simulink model "dofAutopilot"  (R2024b)
settings: Solver=ode4  StartTime=0.0  StopTime=10  FixedStep=0.001  MaxStep=0.2  RelTol=1e-3
libraries: slpidlib x2, shared6dof x1, aerolibatmos2 x1
settings Model: Creator=sahil  LastModifiedBy=sahil

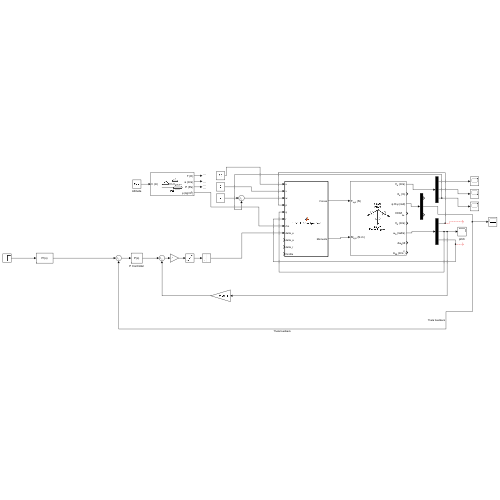
[thumbnail: Simulink's stored preview of the top-level diagram]
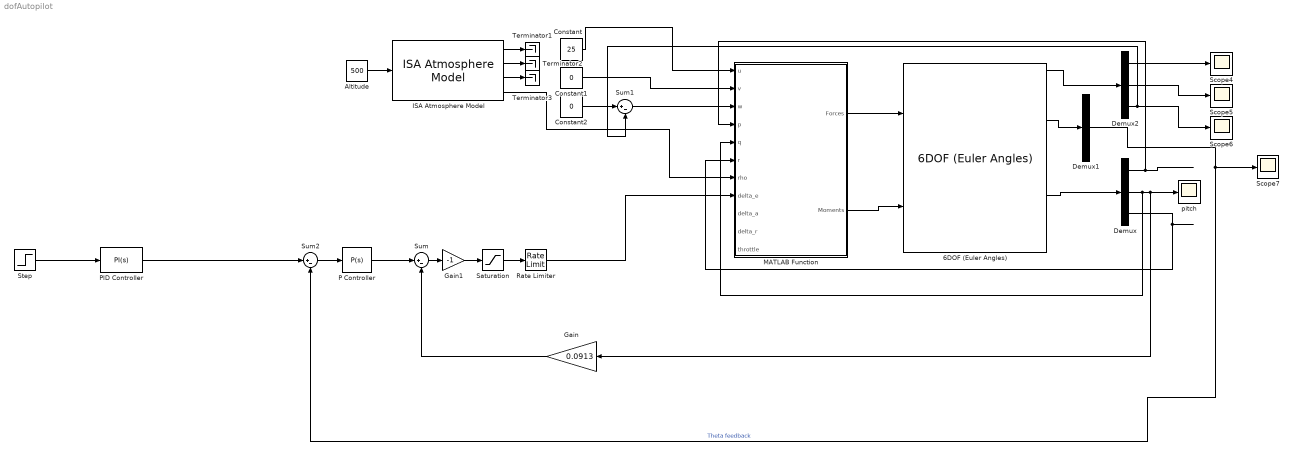
== system dofAutopilot ==
  6DOF (Euler Angles) : shared6dof/6DOF (Euler Angles)  units=Metric (MKS)  mtype=Fixed  rep=Euler Angles  xme_0=[0 0 0]  Vm_0=[15 0 0]  eul_0=[0 0 0]  pm_0=[0 0 0]  mass_0=13.5  mass_e=0.5  mass_f=2.0  inertia=[0.824 0 0.120; 0 1.135 0; 0.120 0 1.759]  inertia_e=eye(3)  inertia_f=2*eye(3)  k_quat=1.0  vre_flag=on  abi_flag=off  aMode=0  xme_statename=''  Vm_statename=''  eul_statename=''  quat_statename=''  pm_statename=''  mass_statename=''
  Altitude : Constant  Value=500
  Constant : Constant  Value=25
  Constant1 : Constant  Value=0
  Constant2 : Constant  Value=0
  Demux : Demux  Outputs=3
  Demux1 : Demux  Outputs=3
  Demux2 : Demux  Outputs=3
  Gain : Gain  Gain=0.0913
  Gain1 : Gain  Gain=-1
  ISA Atmosphere Model : aerolibatmos2/ISA Atmosphere Model  useExtended=off  action=Warning  custom=off  viscosityOut=off  g=9.80665  gamma=1.4  R=287.0531  L=0.0065  h_trop=11000  h_strat=20000  rho0=1.225  P0=101325  T0=288.15  h0=0  S=110.4  Tref=273.15  muref=1.716e-5
  MATLAB Function : MATLAB Function  TreatAsAtomicUnit=on
  P Controller : slpidlib/PID Controller  Controller=P  Form=Parallel  TimeDomain=Continuous-time  UseExternalTs=off  SampleTime=-1  IntegratorMethod=Forward Euler  FilterMethod=Forward Euler  ControllerParametersSource=internal  P=1.01058981940052  I=0  UseKiTs=off  D=0  UseExternalDerivativeSource=off  N=100  UseFilter=on  TunerSelectOption=Transfer Function Based (PID Tuner App)  InitialConditionSource=internal  InitialConditionForIntegrator=0  InitialConditionForFilter=0  DifferentiatorICPrevScaledInput=0  ExternalReset=none  TrackingMode=off  Kt=1  LimitOutput=off  SatLimitsSource=internal  UpperSaturationLimit=inf  LowerSaturationLimit=-inf  LinearizeAsGain=on  AntiWindupMode=none  Kb=1  LimitIntegrator=off  UpperIntegratorSaturationLimit=inf  LowerIntegratorSaturationLimit=-inf  POutMin=[]  POutMax=[]  IOutMin=[]  IOutMax=[]  DOutMin=[]  DOutMax=[]  NOutMin=[]  NOutMax=[]  SumOutMin=[]  SumOutMax=[]  SaturationOutMin=[]  SaturationOutMax=[]  PParamMin=[]  PParamMax=[]  IParamMin=[]  IParamMax=[]  DParamMin=[]  DParamMax=[]  NParamMin=[]  NParamMax=[]  KbParamMin=[]  KbParamMax=[]  KtParamMin=[]  KtParamMax=[]  KbOutMin=[]  KbOutMax=[]  KtOutMin=[]  KtOutMax=[]  IntegratorOutMin=[]  IntegratorOutMax=[]  FilterOutMin=[]  FilterOutMax=[]  SumI1OutMin=[]  SumI1OutMax=[]  SumI2OutMin=[]  SumI2OutMax=[]  SumI3OutMin=[]  SumI3OutMax=[]  SumI4OutMin=[]  SumI4OutMax=[]  SumDOutMin=[]  SumDOutMax=[]  DifferentiatorOutMin=[]  DifferentiatorOutMax=[]  FilterDiffOutCoefMin=[]  FilterDiffOutCoefMax=[]  ReciprocalOutMin=[]  ReciprocalOutMax=[]  SumDenOutMin=[]  SumDenOutMax=[]  SumNumOutMin=[]  SumNumOutMax=[]  DivideOutMin=[]  DivideOutMax=[]  UdiffTsProdOutMin=[]  UdiffTsProdOutMax=[]  NTsProdOutMin=[]  NTsProdOutMax=[]  UintegralTsProdOutMin=[]  UintegralTsProdOutMax=[]  UngainTsProdOutMin=[]  UngainTsProdOutMax=[]  ClampingZeroOutDataTypeStr=Inherit: Inherit via back propagation  ClampingZeroOutMin=[]  ClampingZeroOutMax=[]  FilterDenConstantOutDataTypeStr=Inherit: Inherit via back propagation  FilterDenConstantOutMin=[]  FilterDenConstantOutMax=[]  PCopyOutDataTypeStr=Inherit: Inherit via back propagation  PCopyOutMin=[]  PCopyOutMax=[]  NCopyOutDataTypeStr=Inherit: Inherit via back propagation  NCopyOutMin=[]  NCopyOutMax=[]  IntegratorContinuousStateAttributes=''  IntegratorStateMustResolveToSignalObject=off  IntegratorRTWStateStorageClass=Auto  FilterContinuousStateAttributes=''  FilterStateMustResolveToSignalObject=off  FilterRTWStateStorageClass=Auto  ParallelPVariant=InternalParameters  IdealPVariant=Disabled  IVariant=Disabled  DVariant=Disabled  IntegratorVariant=Disabled  SatVariant=Disabled  AWVariant=Disabled  PCopyVariant=Disabled  TRVariant=Disabled  FdbkBlocksVariant=Forward  IdealPFdbkVariant=Disabled  SatFdbkVariant=Disabled  DerivativeFilterVariant=Disabled  NVariant=Disabled  NCopyVariant=Disabled_SignalSpec  FilterICVariant=Disabled  IntegratorICVariant=Disabled  ExternalResetVariant=Disabled  TRSumVariant=Passthrough  SumFdbkVariant=Disabled  SumVariant=Passthrough_P  TsampFilterVariant=InternalTs  TsampNgainVariant=Passthrough  TsampIntegralVariant=Disabled_SignalSpec  ExternalSaturationOutDataTypeStr=Inherit: Same as second input  DerivativeSourceVariant=Disabled  PreIntVariant=InternalPreInt
  PID Controller : slpidlib/PID Controller  Controller=PI  Form=Parallel  TimeDomain=Continuous-time  UseExternalTs=off  SampleTime=-1  IntegratorMethod=Forward Euler  FilterMethod=Forward Euler  ControllerParametersSource=internal  P=0.00302835474355919  I=0.00038250519229473  UseKiTs=off  D=0  UseExternalDerivativeSource=off  N=100  UseFilter=on  TunerSelectOption=Transfer Function Based (PID Tuner App)  InitialConditionSource=internal  InitialConditionForIntegrator=0  InitialConditionForFilter=0  DifferentiatorICPrevScaledInput=0  ExternalReset=none  TrackingMode=off  Kt=1  LimitOutput=off  SatLimitsSource=internal  UpperSaturationLimit=inf  LowerSaturationLimit=-inf  LinearizeAsGain=on  AntiWindupMode=none  Kb=1  LimitIntegrator=off  UpperIntegratorSaturationLimit=inf  LowerIntegratorSaturationLimit=-inf  POutMin=[]  POutMax=[]  IOutMin=[]  IOutMax=[]  DOutMin=[]  DOutMax=[]  NOutMin=[]  NOutMax=[]  SumOutMin=[]  SumOutMax=[]  SaturationOutMin=[]  SaturationOutMax=[]  PParamMin=[]  PParamMax=[]  IParamMin=[]  IParamMax=[]  DParamMin=[]  DParamMax=[]  NParamMin=[]  NParamMax=[]  KbParamMin=[]  KbParamMax=[]  KtParamMin=[]  KtParamMax=[]  KbOutMin=[]  KbOutMax=[]  KtOutMin=[]  KtOutMax=[]  IntegratorOutMin=[]  IntegratorOutMax=[]  FilterOutMin=[]  FilterOutMax=[]  SumI1OutMin=[]  SumI1OutMax=[]  SumI2OutMin=[]  SumI2OutMax=[]  SumI3OutMin=[]  SumI3OutMax=[]  SumI4OutMin=[]  SumI4OutMax=[]  SumDOutMin=[]  SumDOutMax=[]  DifferentiatorOutMin=[]  DifferentiatorOutMax=[]  FilterDiffOutCoefMin=[]  FilterDiffOutCoefMax=[]  ReciprocalOutMin=[]  ReciprocalOutMax=[]  SumDenOutMin=[]  SumDenOutMax=[]  SumNumOutMin=[]  SumNumOutMax=[]  DivideOutMin=[]  DivideOutMax=[]  UdiffTsProdOutMin=[]  UdiffTsProdOutMax=[]  NTsProdOutMin=[]  NTsProdOutMax=[]  UintegralTsProdOutMin=[]  UintegralTsProdOutMax=[]  UngainTsProdOutMin=[]  UngainTsProdOutMax=[]  ClampingZeroOutDataTypeStr=Inherit: Inherit via back propagation  ClampingZeroOutMin=[]  ClampingZeroOutMax=[]  FilterDenConstantOutDataTypeStr=Inherit: Inherit via back propagation  FilterDenConstantOutMin=[]  FilterDenConstantOutMax=[]  PCopyOutDataTypeStr=Inherit: Inherit via back propagation  PCopyOutMin=[]  PCopyOutMax=[]  NCopyOutDataTypeStr=Inherit: Inherit via back propagation  NCopyOutMin=[]  NCopyOutMax=[]  IntegratorContinuousStateAttributes=''  IntegratorStateMustResolveToSignalObject=off  IntegratorRTWStateStorageClass=Auto  FilterContinuousStateAttributes=''  FilterStateMustResolveToSignalObject=off  FilterRTWStateStorageClass=Auto  ParallelPVariant=InternalParameters  IdealPVariant=Disabled  IVariant=InternalParameters  DVariant=Disabled  IntegratorVariant=Continuous  SatVariant=Disabled  AWVariant=Passthrough  PCopyVariant=Disabled  TRVariant=Disabled  FdbkBlocksVariant=Forward  IdealPFdbkVariant=Disabled  SatFdbkVariant=Disabled  DerivativeFilterVariant=Disabled  NVariant=Disabled  NCopyVariant=Disabled_SignalSpec  FilterICVariant=Disabled  IntegratorICVariant=InternalICs  ExternalResetVariant=Disabled  TRSumVariant=Passthrough  SumFdbkVariant=Disabled  SumVariant=Sum_PI  TsampFilterVariant=InternalTs  TsampNgainVariant=Passthrough  TsampIntegralVariant=Disabled_SignalSpec  ExternalSaturationOutDataTypeStr=Inherit: Same as second input  DerivativeSourceVariant=Disabled  PreIntVariant=InternalPreInt
  Rate Limiter : RateLimiter  RisingSlewLimit=45*pi/180  FallingSlewLimit=-45*pi/180  SampleTimeMode=inherited
  Saturation : Saturate  UpperLimit=25*pi/180  LowerLimit=-25*pi/180
  Scope{4..7} (4 alike) : Scope
  Step : Step  After=5/57.3  SampleTime=0
  Sum : Sum  Inputs=|+-
  Sum1 : Sum  Inputs=|+-
  Sum2 : Sum  Inputs=|+-
  Terminator1 : Terminator
  Terminator2 : Terminator
  Terminator3 : Terminator
  pitch : Scope
  wires:
  Altitude/1 -> ISA Atmosphere Model/1
  ISA Atmosphere Model/1 -> Terminator1/1
  ISA Atmosphere Model/2 -> Terminator2/1
  ISA Atmosphere Model/3 -> Terminator3/1
  ISA Atmosphere Model/4 -> MATLAB Function/7(rho)
  MATLAB Function/1(Forces) -> 6DOF (Euler Angles)/1
  MATLAB Function/2(Moments) -> 6DOF (Euler Angles)/2
  6DOF (Euler Angles)/1 -> Demux2/1
  6DOF (Euler Angles)/6 -> Demux/1
  Demux/1 -> MATLAB Function/4(p)
  Demux/3 -> MATLAB Function/6(r)
  Demux2/1 -> Scope4/1
  Demux2/2 -> Scope5/1
  Demux2/3 -> Sum1/2, Scope6/1
  Constant/1 -> MATLAB Function/1(u)
  Constant1/1 -> MATLAB Function/2(v)
  Constant2/1 -> Sum1/1
  Sum1/1 -> MATLAB Function/3(w)
  6DOF (Euler Angles)/3 -> Demux1/1
  Gain1/1 -> Saturation/1
  PID Controller/1 -> Sum2/1
  Step/1 -> PID Controller/1
  Saturation/1 -> Rate Limiter/1
  Sum/1 -> Gain1/1
  Gain/1 -> Sum/2
  Rate Limiter/1 -> MATLAB Function/8(delta_e)
  Sum2/1 -> P Controller/1
  Demux1/2 -> Sum2/2, Scope7/1  "Theta feedback"
  P Controller/1 -> Sum/1
  Demux/2 -> MATLAB Function/5(q), Gain/1, pitch/1

== matlab function dofAutopilot/MATLAB Function ==
  data: u input; Forces output; v input; w input; p input; q input; r input; rho input; Moments output; delta_e input; delta_a input; delta_r input; throttle input
function [Forces, Moments] = computeAeroDynamics(u, v, w, p, q, r, rho, delta_e, delta_a, delta_r, throttle)
% Inputs:
% u, v, w  - Body frame velocities in m/s
% p, q, r  - Body frame angular rates in rad/s
% rho      - Air density in kg/m^3
% delta_e  - Elevator deflection in radians
% delta_a  - Aileron deflection in radians
% delta_r  - Rudder deflection in radians
% throttle - Throttle command (0 to 1)

    %% 1. Aircraft Geometry & Reference Values (Aerosonde UAV)
    S = 0.55;         % Reference wing area (m^2)
    b = 2.895;        % Wingspan (m)
    c_bar = 0.1899;   % Mean aerodynamic chord (m)
    
    %% 2. Airflow Angles & Dynamic Pressure
    V = sqrt(u^2 + v^2 + w^2);
    V_safe = max(V, 0.1); 
    
    alpha = atan2(w, u);
    beta = asin(v / V_safe);
    
    q_bar = 0.5 * rho * V^2; % Dynamic pressure
    
    %% 3. Aerodynamic Stability Derivatives (Aerosonde Standards)
    % Longitudinal Derivatives
    CL0 = 0.28;      CLa = 5.61;      CLq = 0;      CLde = 0.13;
    CD0 = 0.03;      K = 0.055;       % Induced drag factor
    Cm0 = -0.02;     Cma = -2.74;     Cmq = -38.21;    Cmde = -2.31; % FIXED: Was -231
    
    % Lateral-Directional Derivatives
    CYb = -0.17;     CYp = 0;         CYr = 0;         CYdr = 0.208;
    Clb = -0.13;     Clp = -0.51;     Clr = 0.265;     Clda = 0.17;   Cldr = 0.045;
    Cnb = 0.073;     Cnp = -0.14;     Cnr = -0.096;    Cnda = 0.0042;  Cndr = -0.069;
    
    %% 4. Non-Dimensional Coefficients
    % Lift, Drag, and Pitch Moment
    CL = CL0 + CLa*alpha + CLq*(q*c_bar/(2*V_safe)) + CLde*delta_e;
    CD = CD0 + K*(CL^2);
    Cm = Cm0 + Cma*alpha + Cmq*(q*c_bar/(2*V_safe)) + Cmde*delta_e;
    
    % Sideforce, Roll, and Yaw Moment
    CY = CYb*beta + CYp*(p*b/(2*V_safe)) + CYr*(r*b/(2*V_safe)) + CYdr*delta_r;
    Cl = Clb*beta + Clp*(p*b/(2*V_safe)) + Clr*(r*b/(2*V_safe)) + Clda*delta_a + Cldr*delta_r;
    Cn = Cnb*beta + Cnp*(p*b/(2*V_safe)) + Cnr*(r*b/(2*V_safe)) + Cnda*delta_a + Cndr*delta_r;
    
    %% 5. Dimensional Aerodynamic Forces (Wind to Body Frame)
    L_aero = q_bar * S * CL;
    D_aero = q_bar * S * CD;
    Y_aero = q_bar * S * CY;
    
    Fx_aero = -D_aero * cos(alpha) + L_aero * sin(alpha);
    Fy_aero = Y_aero;
    Fz_aero = -D_aero * sin(alpha) - L_aero * cos(alpha);
    
    %% 6. Dimensional Aerodynamic Moments
    L_moment = q_bar * S * b * Cl;
    M_moment = q_bar * S * c_bar * Cm;
    N_moment = q_bar * S * b * Cn;
    
    %% 7. Propulsion Model
    % Realistic thrust for a 13.5kg UAV (approx 80N max)
    max_thrust = 80; 
    Thrust = max_thrust * throttle;
    
    Fx_total = Fx_aero + Thrust;
    Fy_total = Fy_aero;
    Fz_total = Fz_aero;
    
    %% 8. Compile Outputs
    Forces = [Fx_total; Fy_total; Fz_total];
    Moments = [L_moment; M_moment; N_moment];
end
